simulink model "ads_simulink"  (R2016a)
settings: Solver=VariableStepAuto  StartTime=0.0  StopTime=10.0  RelTol=1e-3
libraries: simulink x2, dspsigops x2
settings Model: Creator=Kendall Kuzminskas  LastModifiedBy=Kendall Kuzminskas

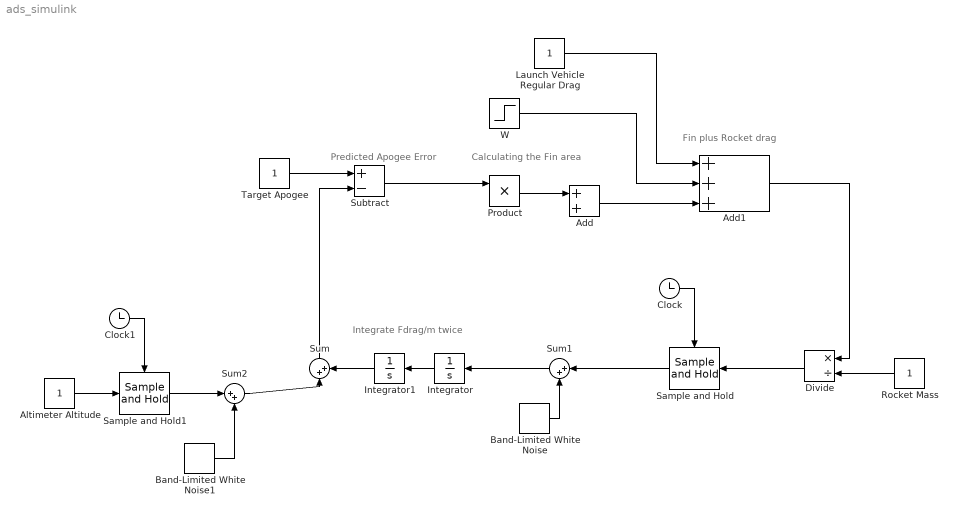
== system ads_simulink ==
  note: Integrate Fdrag/m twice
  note: Fin plus Rocket drag
  note: Predicted Apogee Error
  note: Calculating the Fin area
  Add : Sum
  Add1 : Sum  Inputs=+++
  Altimeter Altitude : Constant
  Band-Limited White Noise : simulink/Sources/Band-Limited White Noise  Cov=[0.1]  Ts=0.1  seed=[23341]
  Band-Limited White Noise1 : simulink/Sources/Band-Limited White Noise  Cov=[0.1]  Ts=0.1  seed=[23341]
  Clock : Clock
  Clock1 : Clock
  Divide : Product  Inputs=*/
  Integrator : Integrator
  Integrator1 : Integrator
  Launch Vehicle Regular Drag : Constant
  Product : Product
  Rocket Mass : Constant
  Sample and Hold : dspsigops/Sample and Hold  trig=Rising edge  initCond=0  latchinput=off
  Sample and Hold1 : dspsigops/Sample and Hold  trig=Rising edge  initCond=0  latchinput=off
  Subtract : Sum  Inputs=+-
  Sum : Sum  Inputs=|++
  Sum1 : Sum  Inputs=|++
  Sum2 : Sum  Inputs=|++
  Target Apogee : Constant
  W : Step  SampleTime=0
  wires:
  Product/1 -> Add/1
  Subtract/1 -> Product/1
  Target Apogee/1 -> Subtract/1
  Add/1 -> Add1/3
  Launch Vehicle Regular Drag/1 -> Add1/1
  W/1 -> Add1/2
  Add1/1 -> Divide/1
  Rocket Mass/1 -> Divide/2
  Divide/1 -> Sample and Hold/1
  Clock/1 -> Sample and Hold/Trigger
  Integrator/1 -> Integrator1/1
  Sum/1 -> Subtract/2
  Band-Limited White Noise/1 -> Sum1/2
  Sample and Hold/1 -> Sum1/1
  Sum1/1 -> Integrator/1
  Band-Limited White Noise1/1 -> Sum2/2
  Sum2/1 -> Sum/1
  Clock1/1 -> Sample and Hold1/Trigger
  Altimeter Altitude/1 -> Sample and Hold1/1
  Sample and Hold1/1 -> Sum2/1
  Integrator1/1 -> Sum/2
